simulink model "altOptMPC_th"  (R2020a)
settings: Solver=VariableStepAuto  StartTime=0.0  StopTime=simTime  RelTol=1e-3
values from neighbouring files (symbols this model uses):
  maxAlt = max(xMeasure)    [altOptMPC_ts.m]
  minAlt = min(xMeasure)    [altOptMPC_ts.m]
libraries: kfgpPrediction x1, mpcgpkf_altitudeOptimization x1, simpleTetheredBalloon x1, syntheticFlowGenerator x1
settings Model: PacingRate=5  Creator=Ayaz  LastModifiedBy=Ayaz

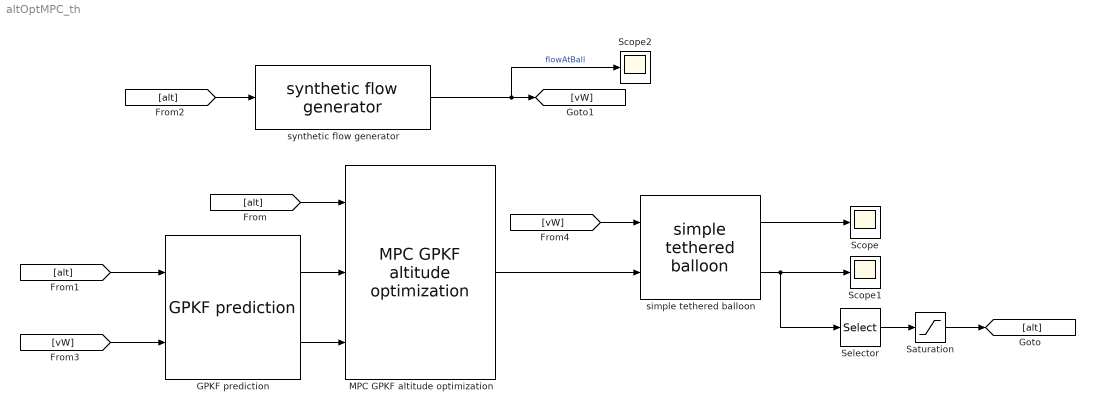
== system altOptMPC_th ==
  GPKF prediction : kfgpPrediction/GPKF prediction  gpkfTimeStep=kfgptimeStep  timeScale=timeScale  spatialScale=altScale  covAmp=covAmp  xMeasure=xMeasure  noiseVar=noiseVar  hTau=tempKern  powerLawParams=powLawParams
  MPC GPKF altitude optimization : mpcgpkf_altitudeOptimization/MPC GPKF altitude optimization  timeScale=timeScale  spatialScale=altScale  covAmp=covAmp  xMeasure=xMeasure  noiseVar=noiseVar  hTau=tempKern  powerLawParams=powLawParams  mpcgpkfTimeStep=mpctimeStep  nPred=nPred  zMax=maxAlt  zMin=minAlt  zStepMax=zStepMax  tradeoffCons=tradeOffCon  iniSP=iniAlt
  Saturation : Saturate  UpperLimit=maxAlt  LowerLimit=minAlt
  Scope : Scope
  Scope1 : Scope
  Scope2 : Scope
  Selector : Selector  InputPortWidth=2  IndexOptions=Index vector (dialog)  Indices=2  OutputSizes=1
  simple tethered balloon : simpleTetheredBalloon/simple tethered balloon  rhoEnv=rhoEnv  rhoBall=rhoBall  rBall=rBall  cdBall=cdBall  kSpring=kThr  iniAlt=iniAlt  kp=altKp  ki=altKi  tau=altTau
  synthetic flow generator : syntheticFlowGenerator/synthetic flow generator  hTau=tempKern  timeScale=timeScale  powerLawParams=powLawParams  tSamp=sampleTimeStep  finalTime=finalTime  stdDev=stdDev  minFlow=minFlowValue  rngSeed=rngSeed  altScale=altScale  covAmp=covAmp  zDiscrete=xMeasure
  wires:
  GPKF prediction/1 -> MPC GPKF altitude optimization/2
  GPKF prediction/2 -> MPC GPKF altitude optimization/3
  MPC GPKF altitude optimization/1 -> simple tethered balloon/2
  simple tethered balloon/1 -> Scope/1
  simple tethered balloon/2 -> Selector/1, Scope1/1
  [alt] -> MPC GPKF altitude optimization/1
  [alt] -> GPKF prediction/1
  synthetic flow generator/1 -> Scope2/1, [vW]  "flowAtBall"
  [vW] -> GPKF prediction/2
  [vW] -> simple tethered balloon/1
  Selector/1 -> Saturation/1
  Saturation/1 -> [alt]
  [alt] -> synthetic flow generator/1
